simulink model "editedopenloop2perfected"  (R2016a)
settings: Solver=VariableStepAuto  StartTime=0.0  StopTime=1  RelTol=1e-3
libraries: powerlib x21, simulink x2, powerlib_meascontrol x1
settings Model: Creator=mojum  LastModifiedBy=mojum

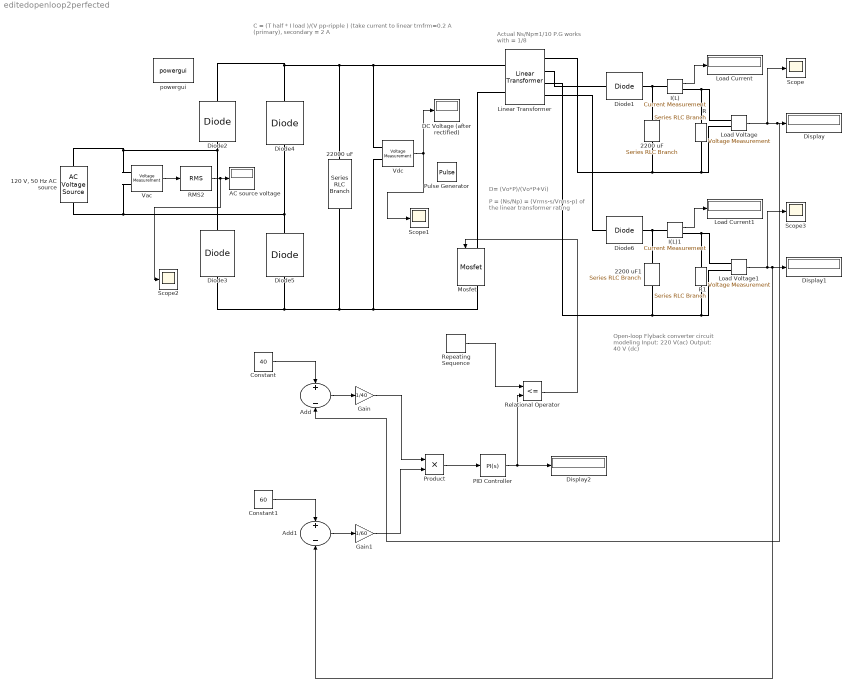
== system editedopenloop2perfected ==
  note: Actual Ns/Np=1/10
      | P.G works with = 1/8
  note: C = (T half * I load )/(V pp-ripple )
      | (take current to linear trnfrm=0.2 A (primary), secondary = 2 A
  note: P = (Ns/Np) = (Vrms-s/Vrms-p)
      | of the linear transformer rating
  note: D= (Vo*P)/(Vo*P+Vi)
  note: Open-loop Flyback
      | converter circuit modeling
      | Input: 220 V(ac)
      | Output: 40 V (dc)
  "120 V, 50 Hz AC source" : powerlib/Electrical Sources/AC Voltage Source  Amplitude=240  Phase=0  Frequency=50  SampleTime=0  Measurements=None  BusType=swing  Pref=10e3  Qref=0  Qmin=-inf  Qmax=+inf
  2200 uF : powerlib/Elements/Series RLC Branch  LConnTagsString=__new0  RConnTagsString=__new0  BranchType=C  Resistance=1  Inductance=1e-3  SetiL0=off  InitialCurrent=0  Capacitance=2200e-6  Setx0=off  InitialVoltage=0  Measurements=None
  2200 uF1 : powerlib/Elements/Series RLC Branch  LConnTagsString=__new0  RConnTagsString=__new0  BranchType=C  Resistance=1  Inductance=1e-3  SetiL0=off  InitialCurrent=0  Capacitance=2200e-6  Setx0=off  InitialVoltage=0  Measurements=None
  22000 uF : powerlib/Elements/Series RLC Branch  LConnTagsString=__new0  RConnTagsString=__new0  BranchType=C  Resistance=1  Inductance=1e-3  SetiL0=off  InitialCurrent=0  Capacitance=22000e-6  Setx0=off  InitialVoltage=0  Measurements=None
  AC source voltage : Display
  Add : Sum  Inputs=+-
  Add1 : Sum  Inputs=+-
  Constant : Constant  Value=40
  Constant1 : Constant  Value=60
  DC Voltage (after rectified) : Display
  Diode{1..6} (6 alike) : powerlib/Power Electronics/Diode  Ron=0.001  Lon=0  Vf=0.8  IC=0  UseSnubber=off  Rs=500  Cs=250e-9  Measurements=off
  Display : Display
  Display1 : Display
  Display2 : Display
  Gain : Gain  Gain=1/40
  Gain1 : Gain  Gain=1/60
  I(L) : powerlib/Measurements/Current Measurement  PhasorSimulation=off  OutputType=Complex  PSBequivalent=0
  I(L)1 : powerlib/Measurements/Current Measurement  PhasorSimulation=off  OutputType=Complex  PSBequivalent=0
  Linear Transformer : powerlib/Elements/Linear Transformer  UNITS=SI  NominalPower=[ 25000 100e3 ]  winding1=[400 0 0]  winding2=[40 0 0]  ThreeWindings=on  winding3=[60 0 0]  RmLm=[1e4 1000e-6]  Measurements=Magnetization current  DataType=on
  Load Current : Display
  Load Current1 : Display
  Load Voltage : powerlib/Measurements/Voltage Measurement  PhasorSimulation=off  OutputType=Complex  PSBequivalent=0
  Load Voltage1 : powerlib/Measurements/Voltage Measurement  PhasorSimulation=off  OutputType=Complex  PSBequivalent=0
  Mosfet : powerlib/Power Electronics/Mosfet  Ron=0.1  Lon=0  Rd=0.01  Vfd=0  IC=0  Rs=1e5  Cs=inf  Measurements=on
  PID Controller : simulink/Continuous/PID Controller  Controller=PI  TimeDomain=Continuous-time  SampleTime=-1  IntegratorMethod=Forward Euler  FilterMethod=Forward Euler  Form=Parallel  UseFilter=on  ControllerParametersSource=internal  P=0.8  I=100  D=10  N=1  InitialConditionSource=internal  InitialConditionForIntegrator=0  InitialConditionForFilter=0  ExternalReset=none  LimitOutput=on  UpperSaturationLimit=.99  LowerSaturationLimit=.1  LinearizeAsGain=on  AntiWindupMode=none  Kb=1  TrackingMode=off  Kt=1  PParamMin=[]  PParamMax=[]  IParamMin=[]  IParamMax=[]  DParamMin=[]  DParamMax=[]  NParamMin=[]  NParamMax=[]  KbParamMin=[]  KbParamMax=[]  KtParamMin=[]  KtParamMax=[]  POutMin=[]  POutMax=[]  IOutMin=[]  IOutMax=[]  DOutMin=[]  DOutMax=[]  NOutMin=[]  NOutMax=[]  KbOutMin=[]  KbOutMax=[]  KtOutMin=[]  KtOutMax=[]  IntegratorOutMin=[]  IntegratorOutMax=[]  FilterOutMin=[]  FilterOutMax=[]  SumOutMin=[]  SumOutMax=[]  SumI1OutMin=[]  SumI1OutMax=[]  SumI2OutMin=[]  SumI2OutMax=[]  SumI3OutMin=[]  SumI3OutMax=[]  SumDOutMin=[]  SumDOutMax=[]  SaturationOutMin=[]  SaturationOutMax=[]  IntegratorContinuousStateAttributes=''  IntegratorStateMustResolveToSignalObject=off  IntegratorRTWStateStorageClass=Auto  FilterContinuousStateAttributes=''  FilterStateMustResolveToSignalObject=off  FilterRTWStateStorageClass=Auto  DifferentiatorICPrevScaledInput=0  DifferentiatorOutMin=[]  DifferentiatorOutMax=[]
  Product : Product
  Pulse Generator : DiscretePulseGenerator  PulseType=Time based  Period=1/100e3  PulseWidth=77
  R : powerlib/Elements/Series RLC Branch  LConnTagsString=__new0  RConnTagsString=__new0  BranchType=R  Resistance=40  Inductance=1e-3  SetiL0=off  InitialCurrent=0  Capacitance=200e-6  Setx0=off  InitialVoltage=0  Measurements=None
  R1 : powerlib/Elements/Series RLC Branch  LConnTagsString=__new0  RConnTagsString=__new0  BranchType=R  Resistance=40  Inductance=1e-3  SetiL0=off  InitialCurrent=0  Capacitance=200e-6  Setx0=off  InitialVoltage=0  Measurements=None
  RMS2 : powerlib_meascontrol/Measurements/RMS  TrueRMS=on  Freq=60  RMSInit=120  Ts=0
  Relational Operator : RelationalOperator  Operator=<=  OutDataTypeStr=boolean
  Repeating Sequence : simulink/Sources/Repeating Sequence  rep_seq_t=[0 1/100000]  rep_seq_y=[0 1]
  Scope{,1..3} (4 alike) : Scope
  Vac : powerlib/Measurements/Voltage Measurement  PhasorSimulation=off  OutputType=Complex  PSBequivalent=0
  "Vdc " : powerlib/Measurements/Voltage Measurement  PhasorSimulation=off  OutputType=Complex  PSBequivalent=0
  powergui : powerlib/powergui  Priority=1  SimulationMode=Discrete  SolverType=Tustin/Backward Euler (TBE)  SampleTime=.5e-6  frequency=60  SPID=on  DisableSnubberDevices=off  DisableRonSwitches=off  DisableVfSwitches=off  SwTol=0  DisplayEquations=off  Interpol=off  ExternalGateDelay=off  methode=off  Ts=10  FunctionMessages=off  echomessages=off  HookPort=off  EnableUseOfTLC=off  x0status=blocks  frequencyindice=0  Pbase=100e6  ErrMax=1e-4  Iterations=50  UnitsV=kV  UnitsW=MW  buscounter=0  RestoreLinks=warning  ResistiveCurrentMeasurement=off  Frange=[0:2:500]  Ylog=off  Xlog=on  ShowGrid=off  save=off  variable=ZData  structure=0  ZoomFFT=off  StartTime=0.0  cycles=1  DisplayStyle=1  fundamental=60  FreqAxis=off  MaxFrequency=1000  frequencyindicesteady=1  RmsSteady=1  display=off
  wires:
  Vac/1 -> RMS2/1
  RMS2/1 -> Scope2/1, AC source voltage/1
  "Vdc "/1 -> Scope1/1, DC Voltage (after rectified)/1
  I(L)/1 -> Load Current/1
  I(L)1/1 -> Load Current1/1
  Constant/1 -> Add/1
  Load Voltage/1 -> Add/2, Display/1, Scope/1
  Add/1 -> Gain/1
  PID Controller/1 -> Relational Operator/2, Display2/1
  Repeating Sequence/1 -> Relational Operator/1
  Relational Operator/1 -> Mosfet/1
  Constant1/1 -> Add1/1
  Load Voltage1/1 -> Display1/1, Add1/2, Scope3/1
  Add1/1 -> Gain1/1
  Gain1/1 -> Product/2
  Gain/1 -> Product/1
  Product/1 -> PID Controller/1
  connections:
  Diode4/RConn1 -- Diode2/RConn1 -- "Vdc "/LConn1 -- Linear Transformer/LConn1 -- 22000 uF/LConn1
  Linear Transformer/LConn2 -- Mosfet/LConn1
  Diode1/LConn1 -- Linear Transformer/RConn2
  Diode1/RConn1 -- 2200 uF/LConn1 -- I(L)/LConn1
  R/RConn1 -- Linear Transformer/RConn1 -- 2200 uF/RConn1 -- Load Voltage/LConn2
  "120 V, 50 Hz AC source"/LConn1 -- Vac/LConn2 -- Diode4/LConn1 -- Diode5/RConn1
  Diode5/LConn1 -- "Vdc "/LConn2 -- Mosfet/RConn1 -- 22000 uF/RConn1 -- Diode3/LConn1
  Vac/LConn1 -- "120 V, 50 Hz AC source"/RConn1 -- Diode2/LConn1 -- Diode3/RConn1
  R/LConn1 -- I(L)/RConn1 -- Load Voltage/LConn1
  I(L)1/LConn1 -- Diode6/RConn1 -- 2200 uF1/LConn1
  Load Voltage1/LConn2 -- R1/RConn1 -- Linear Transformer/RConn3 -- 2200 uF1/RConn1
  Load Voltage1/LConn1 -- R1/LConn1 -- I(L)1/RConn1
  Diode6/LConn1 -- Linear Transformer/RConn4
